simulink model "visual_line_follower_with_debug_real"  (R2026a)
settings: Solver=FixedStepDiscrete  StopTime=inf  FixedStep=Ts_Control  EnableMultiTasking=on
InitFcn:
  | run(fullfile(fileparts(get_param(bdroot,"FileName")),"runtime","init","configure_visual_line_follower_real_debug.m"));
model workspace (MAT data in the model file):
  BaseLinearSpeed = 5
  BaseSpeedScale = 0.03
  Kd_Line = 0.35
  Ki_Line = 0
  Kp_Line = 5
  LocalPath_CurvatureGain = 0.04
  LocalPath_HeadingGain = 0.35
  LocalPath_LateralGain = 0.6
  LocalPath_LookaheadDistance = 0.2
  LocalPath_NumPoints = 30
  LocalPath_ROIFraction = 0.1
  MJ_StepTime = 0.002
  MJ_TargetLateralPosition = 0
  MaxAngularSpeed = 1.5
  MaxWheelSpeed = 7.9
  N_Line = 20
  OriginBot_ErrorScale = 500
  OriginBot_MaxSaturation = 0.3
  OriginBot_MinBrightness = 70
  OriginBot_MinPixels = 30
  OriginBot_ROIHeight = 45
  OriginBot_ROIStartFraction = 0.72
  SL_ROS_VariableLengthArrays_MaxSizes.CommonInfo.ArrayTruncateAction = 'EmitWarning'
  SL_ROS_VariableLengthArrays_MaxSizes.MsgTypeMap = containers.Map
  SL_ROS_VariableLengthArrays_MaxSizes.MsgTypeMap.serialization.keys = {'sensor_msgs/Image'}
  SL_ROS_VariableLengthArrays_MaxSizes.MsgTypeMap.serialization.values{1}(1).PropertyName = 'data'
  SL_ROS_VariableLengthArrays_MaxSizes.MsgTypeMap.serialization.values{1}(1).DataType = 'uint8'
  SL_ROS_VariableLengthArrays_MaxSizes.MsgTypeMap.serialization.values{1}(1).MaxLength = 6220800
  SL_ROS_VariableLengthArrays_MaxSizes.MsgTypeMap.serialization.values{1}(2).PropertyName = 'encoding'
  SL_ROS_VariableLengthArrays_MaxSizes.MsgTypeMap.serialization.values{1}(2).DataType = 'uint8'
  SL_ROS_VariableLengthArrays_MaxSizes.MsgTypeMap.serialization.values{1}(2).MaxLength = 128
  SL_ROS_VariableLengthArrays_MaxSizes.MsgTypeMap.serialization.uniformity = 0
  SL_ROS_VariableLengthArrays_MaxSizes.MsgTypeMap.serialization.keyType = 'char'
  SL_ROS_VariableLengthArrays_MaxSizes.MsgTypeMap.serialization.valueType = 'any'
  SteeringSign = 1
  TB3_WheelRadius = 0.033
  TB3_WheelSeparation = 0.16
  Ts_Control = 0.05
  Ts_Vision = 0.05
  TurtleBot3MuJoCoMap = 'simple'
  TurtleBot3MuJoCoScene = ""
  k_heading = 0.55
undefined symbols (not defined in the file or in its folder): originbot_line_follower_debug_frame, originbot_sliding_window_path_generator, twist
libraries: ros2lib x4, slpidlib x1
settings Model: ExtModeTrigDuration=10000  Creator=HP  LastModifiedBy=kevin
settings SolverCC: PositivePriorityOrder=on
settings ConfigComp: CovMetricSettings=dswe

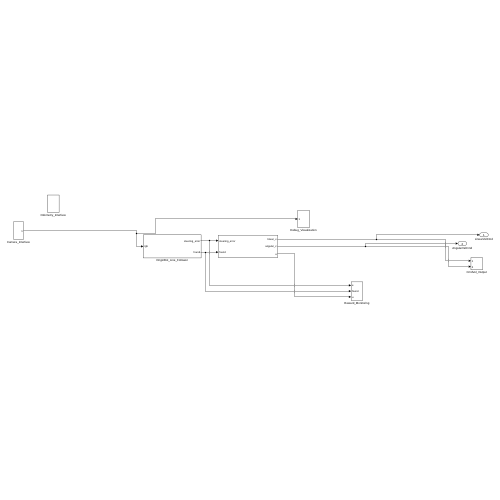
[thumbnail: Simulink's stored preview of the top-level diagram]
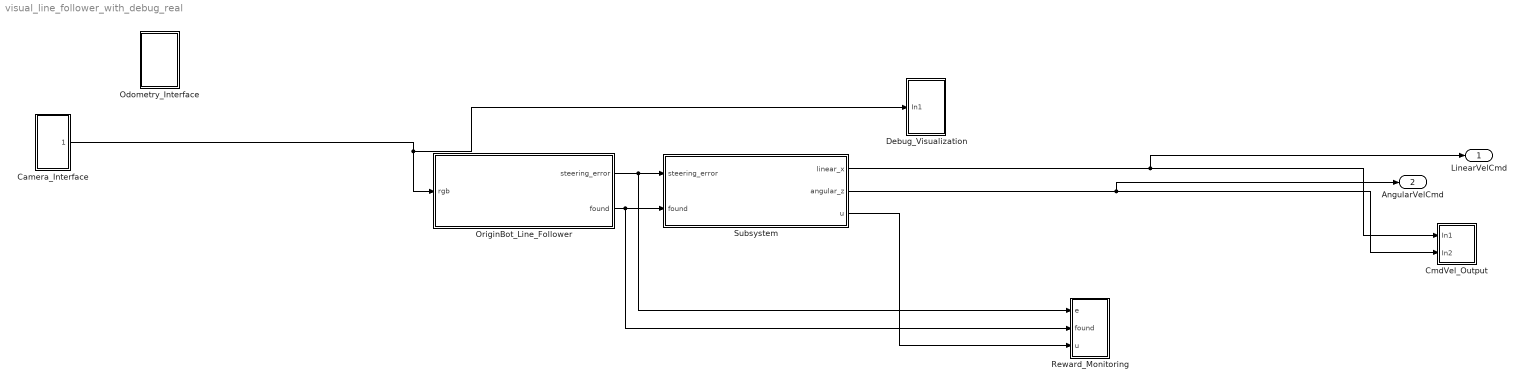
== system visual_line_follower_with_debug_real ==
  Camera_Interface : Subsystem
  CmdVel_Output : Subsystem
  Debug_Visualization : Subsystem
  Odometry_Interface : Subsystem
  OriginBot_Line_Follower : Subsystem
  Reward_Monitoring : Subsystem
  Subsystem : Subsystem
  LinearVelCmd : Outport
  AngularVelCmd : Outport  Port=2
  wires:
  Subsystem/1(linear_x) -> CmdVel_Output/1(In1), LinearVelCmd/1
  Subsystem/2(angular_z) -> CmdVel_Output/2(In2), AngularVelCmd/1
  OriginBot_Line_Follower/1(steering_error) -> Reward_Monitoring/1(e), Subsystem/1(steering_error)
  OriginBot_Line_Follower/2(found) -> Reward_Monitoring/2(found), Subsystem/2(found)
  Camera_Interface/1(Out1) -> Debug_Visualization/1(In1), OriginBot_Line_Follower/1(rgb)
  Subsystem/3(u) -> Reward_Monitoring/3(u)

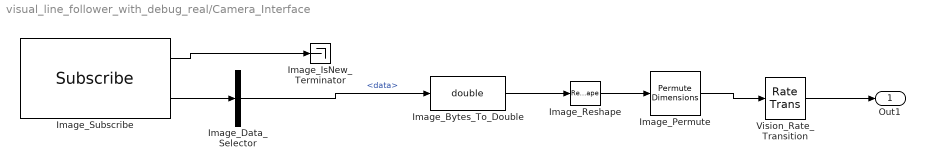
== system visual_line_follower_with_debug_real/Camera_Interface ==
  Image_Bytes_To_Double : DataTypeConversion  OutDataTypeStr=double
  Image_Data_Selector : BusSelector  OutputSignals=data
  Image_IsNew_Terminator : Terminator
  Image_Permute : PermuteDimensions  Order=[3 2 1]
  Image_Reshape : Reshape  OutputDimensionality=Customize  OutputDimensions=[3,1920,1080]
  Image_Subscribe : ros2lib/Subscribe  topicSource=Select from ROS network  topic=/camera/image_raw  messageType=sensor_msgs/Image  sampleTime=Ts_Vision  QOSHistory=Keep last  QOSDepth=10  QOSReliability=Reliable  QOSDurability=Volatile  QOSDeadline=Inf  QOSLifespan=Inf  QOSLiveliness=Automatic  QOSLeaseDuration=Inf  QOSAvoidROSNamespaceConventions=off
  Vision_Rate_Transition : RateTransition
  Out1 : Outport
  wires:
  Image_Permute/1 -> Vision_Rate_Transition/1
  Image_Subscribe/2 -> Image_Data_Selector/1
  Image_Subscribe/1 -> Image_IsNew_Terminator/1
  Image_Data_Selector/1 -> Image_Bytes_To_Double/1  "<data>"
  Vision_Rate_Transition/1 -> Out1/1
  Image_Bytes_To_Double/1 -> Image_Reshape/1
  Image_Reshape/1 -> Image_Permute/1

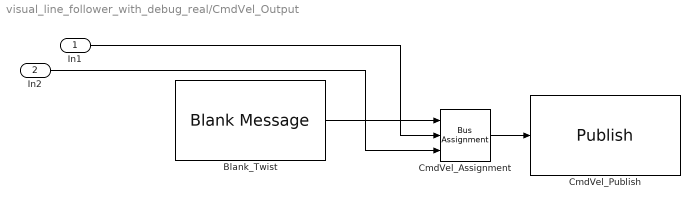
== system visual_line_follower_with_debug_real/CmdVel_Output ==
  In1 : Inport
  In2 : Inport  Port=2
  Blank_Twist : ros2lib/Blank Message  messageClass=Message  entityType=geometry_msgs/TwistStamped  messageType=geometry_msgs/TwistStamped  SampleTime=inf
  CmdVel_Assignment : BusAssignment  AssignedSignals=twist.linear.x,twist.angular.z
  CmdVel_Publish : ros2lib/Publish  topicSource=Select from ROS network  topic=/cmd_vel  messageType=geometry_msgs/TwistStamped  QOSHistory=Keep last  QOSDepth=10  QOSReliability=Reliable  QOSDurability=Volatile  QOSDeadline=Inf  QOSLifespan=Inf  QOSLiveliness=Automatic  QOSLeaseDuration=Inf  QOSAvoidROSNamespaceConventions=off
  wires:
  In2/1 -> CmdVel_Assignment/3
  Blank_Twist/1 -> CmdVel_Assignment/1
  CmdVel_Assignment/1 -> CmdVel_Publish/1
  In1/1 -> CmdVel_Assignment/2

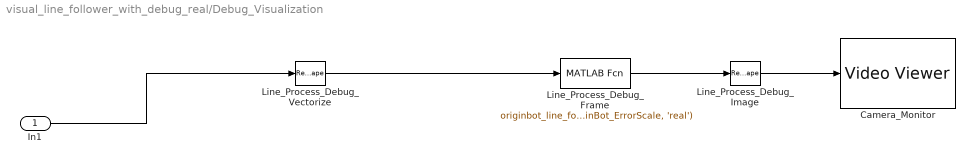
== system visual_line_follower_with_debug_real/Debug_Visualization ==
  In1 : Inport
  Camera_Monitor : VideoViewer  FigPos=[751 777 651 427]
  Line_Process_Debug_Frame : MATLABFcn  MATLABFcn=originbot_line_follower_debug_frame(u, LocalPath_ROIFraction, LocalPath_NumPoints, OriginBot_MinBrightness, OriginBot_MaxSaturation, OriginBot_MinPixels, OriginBot_ErrorScale, 'real')
  Line_Process_Debug_Image : Reshape  OutputDimensionality=Customize  OutputDimensions=[1080,1920,3]
  Line_Process_Debug_Vectorize : Reshape  OutputDimensionality=Column vector (2-D)
  wires:
  Line_Process_Debug_Vectorize/1 -> Line_Process_Debug_Frame/1
  Line_Process_Debug_Image/1 -> Camera_Monitor/1
  Line_Process_Debug_Frame/1 -> Line_Process_Debug_Image/1
  In1/1 -> Line_Process_Debug_Vectorize/1

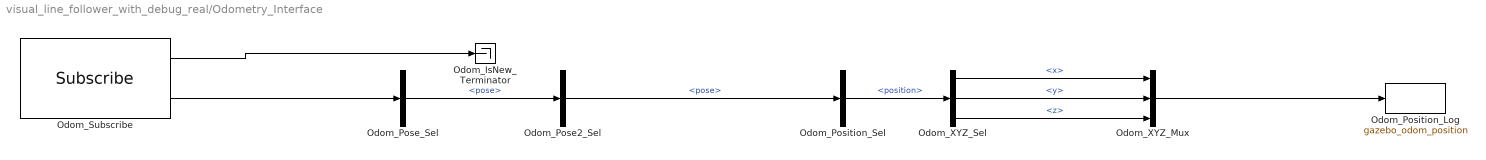
== system visual_line_follower_with_debug_real/Odometry_Interface ==
  Odom_IsNew_Terminator : Terminator
  Odom_Pose2_Sel : BusSelector  OutputSignals=pose
  Odom_Pose_Sel : BusSelector  OutputSignals=pose
  Odom_Position_Log : ToWorkspace  VariableName=gazebo_odom_position  SaveFormat=Timeseries  SampleTime=-1
  Odom_Position_Sel : BusSelector  OutputSignals=position
  Odom_Subscribe : ros2lib/Subscribe  topicSource=Select from ROS network  topic=/odom  messageType=nav_msgs/Odometry  sampleTime=Ts_Control  QOSHistory=Keep last  QOSDepth=10  QOSReliability=Reliable  QOSDurability=Volatile  QOSDeadline=Inf  QOSLifespan=Inf  QOSLiveliness=Automatic  QOSLeaseDuration=Inf  QOSAvoidROSNamespaceConventions=off
  Odom_XYZ_Mux : Mux  Inputs=3
  Odom_XYZ_Sel : BusSelector  OutputSignals=x,y,z
  wires:
  Odom_Subscribe/1 -> Odom_IsNew_Terminator/1
  Odom_XYZ_Sel/3 -> Odom_XYZ_Mux/3  "<z>"
  Odom_Position_Sel/1 -> Odom_XYZ_Sel/1  "<position>"
  Odom_XYZ_Sel/1 -> Odom_XYZ_Mux/1  "<x>"
  Odom_XYZ_Sel/2 -> Odom_XYZ_Mux/2  "<y>"
  Odom_Pose_Sel/1 -> Odom_Pose2_Sel/1  "<pose>"
  Odom_Subscribe/2 -> Odom_Pose_Sel/1
  Odom_Pose2_Sel/1 -> Odom_Position_Sel/1  "<pose>"
  Odom_XYZ_Mux/1 -> Odom_Position_Log/1

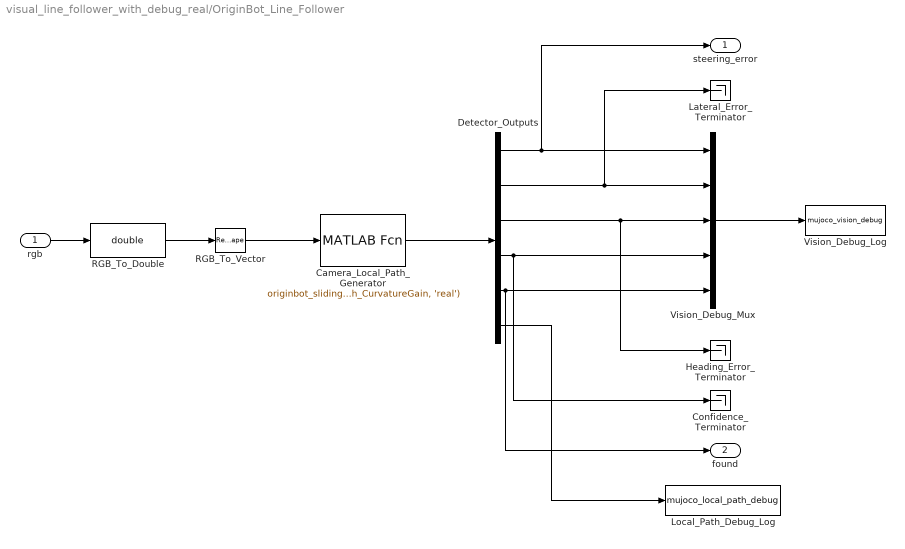
== system visual_line_follower_with_debug_real/OriginBot_Line_Follower ==
  rgb : Inport
  Camera_Local_Path_Generator : MATLABFcn  MATLABFcn=originbot_sliding_window_path_generator(u, LocalPath_ROIFraction, LocalPath_NumPoints, OriginBot_MinBrightness, OriginBot_MaxSaturation, OriginBot_MinPixels, OriginBot_ErrorScale, LocalPath_LookaheadDistance, LocalPath_LateralGain, LocalPath_HeadingGain, LocalPath_CurvatureGain, 'real')  OutputDimensions=72  OutputSignalType=real  SampleTime=Ts_Vision
  Confidence_Terminator : Terminator
  Detector_Outputs : Demux  Outputs=[1 1 1 1 1 67]
  Heading_Error_Terminator : Terminator
  Lateral_Error_Terminator : Terminator
  Local_Path_Debug_Log : ToWorkspace  VariableName=mujoco_local_path_debug  SaveFormat=Timeseries  SampleTime=-1
  RGB_To_Double : DataTypeConversion  OutDataTypeStr=double
  RGB_To_Vector : Reshape  OutputDimensionality=Column vector (2-D)
  Vision_Debug_Log : ToWorkspace  VariableName=mujoco_vision_debug  SaveFormat=Timeseries  SampleTime=-1
  Vision_Debug_Mux : Mux  Inputs=5
  steering_error : Outport
  found : Outport  Port=2
  wires:
  Vision_Debug_Mux/1 -> Vision_Debug_Log/1
  Detector_Outputs/1 -> steering_error/1, Vision_Debug_Mux/1
  Detector_Outputs/5 -> Vision_Debug_Mux/5, found/1
  Detector_Outputs/2 -> Vision_Debug_Mux/2, Lateral_Error_Terminator/1
  Detector_Outputs/6 -> Local_Path_Debug_Log/1
  Detector_Outputs/3 -> Vision_Debug_Mux/3, Heading_Error_Terminator/1
  Detector_Outputs/4 -> Confidence_Terminator/1, Vision_Debug_Mux/4
  RGB_To_Double/1 -> RGB_To_Vector/1
  RGB_To_Vector/1 -> Camera_Local_Path_Generator/1
  rgb/1 -> RGB_To_Double/1
  Camera_Local_Path_Generator/1 -> Detector_Outputs/1

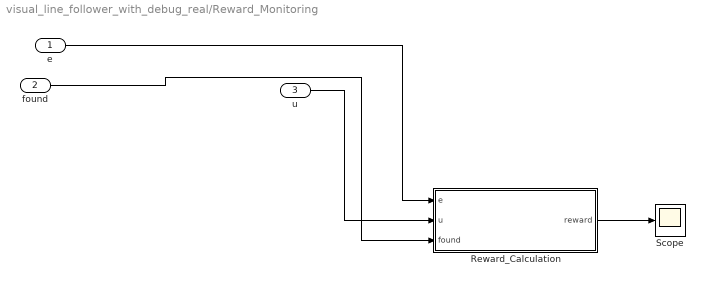
== system visual_line_follower_with_debug_real/Reward_Monitoring ==
  e : Inport
  found : Inport  Port=2
  u : Inport  Port=3
  Reward_Calculation : Subsystem
  Scope : Scope
      settings: ActiveDisplayYMinimum=-19.654077355148576  ActiveDisplayYMaximum=1.5094488795252738
  wires:
  Reward_Calculation/1(reward) -> Scope/1
  u/1 -> Reward_Calculation/2(u)
  e/1 -> Reward_Calculation/1(e)
  found/1 -> Reward_Calculation/3(found)

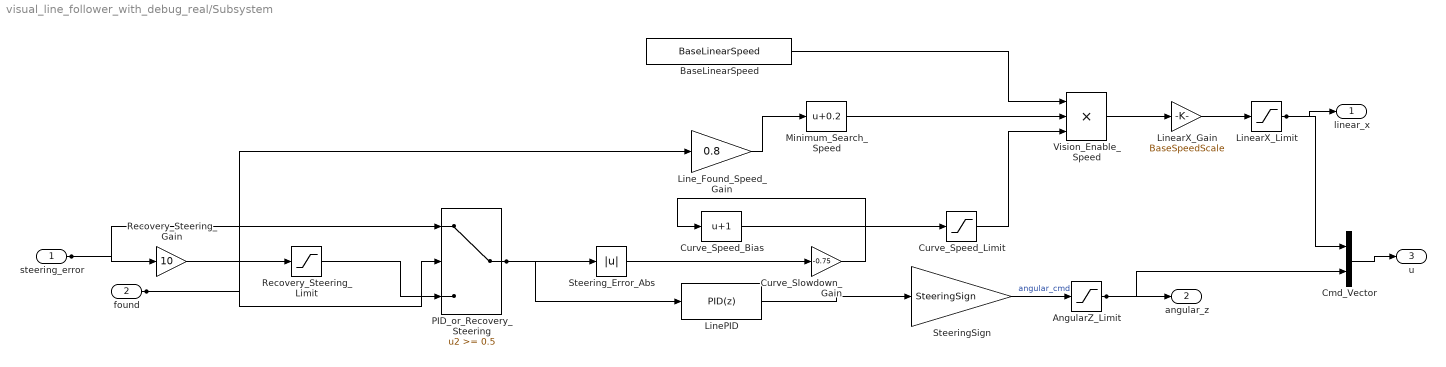
== system visual_line_follower_with_debug_real/Subsystem ==
  steering_error : Inport
  found : Inport  Port=2
  AngularZ_Limit : Saturate  UpperLimit=2*MaxWheelSpeed*TB3_WheelRadius/TB3_WheelSeparation  LowerLimit=-2*MaxWheelSpeed*TB3_WheelRadius/TB3_WheelSeparation
  BaseLinearSpeed : Constant  Value=BaseLinearSpeed
  Cmd_Vector : Mux  Inputs=2
  Curve_Slowdown_Gain : Gain  Gain=-0.75
  Curve_Speed_Bias : Bias  Bias=1
  Curve_Speed_Limit : Saturate  UpperLimit=1  LowerLimit=0.25
  LinePID : slpidlib/PID Controller  Controller=PID  Form=Parallel  TimeDomain=Discrete-time  UseExternalTs=off  SampleTime=Ts_Control  IntegratorMethod=Backward Euler  FilterMethod=Trapezoidal  ControllerParametersSource=internal  P=Kp_Line  I=Ki_Line  UseKiTs=off  D=Kd_Line  UseExternalDerivativeSource=off  N=N_Line  UseFilter=on  TunerSelectOption=Transfer Function Based (PID Tuner App)  InitialConditionSource=internal  InitialConditionForIntegrator=0  InitialConditionForFilter=0  DifferentiatorICPrevScaledInput=0  ExternalReset=none  TrackingMode=off  Kt=1  LimitOutput=on  SatLimitsSource=internal  UpperSaturationLimit=MaxAngularSpeed  LowerSaturationLimit=-MaxAngularSpeed  LinearizeAsGain=off  AntiWindupMode=back-calculation  Kb=1  LimitIntegrator=off  UpperIntegratorSaturationLimit=inf  LowerIntegratorSaturationLimit=-inf  POutMin=[]  POutMax=[]  IOutMin=[]  IOutMax=[]  DOutMin=[]  DOutMax=[]  NOutMin=[]  NOutMax=[]  SumOutMin=[]  SumOutMax=[]  SaturationOutMin=[]  SaturationOutMax=[]  PParamMin=[]  PParamMax=[]  IParamMin=[]  IParamMax=[]  DParamMin=[]  DParamMax=[]  NParamMin=[]  NParamMax=[]  KbParamMin=[]  KbParamMax=[]  KtParamMin=[]  KtParamMax=[]  KbOutMin=[]  KbOutMax=[]  KtOutMin=[]  KtOutMax=[]  IntegratorOutMin=[]  IntegratorOutMax=[]  FilterOutMin=[]  FilterOutMax=[]  SumI1OutMin=[]  SumI1OutMax=[]  SumI2OutMin=[]  SumI2OutMax=[]  SumI3OutMin=[]  SumI3OutMax=[]  SumI4OutMin=[]  SumI4OutMax=[]  SumDOutMin=[]  SumDOutMax=[]  DifferentiatorOutMin=[]  DifferentiatorOutMax=[]  FilterDiffOutCoefMin=[]  FilterDiffOutCoefMax=[]  ReciprocalOutMin=[]  ReciprocalOutMax=[]  SumDenOutMin=[]  SumDenOutMax=[]  SumNumOutMin=[]  SumNumOutMax=[]  DivideOutMin=[]  DivideOutMax=[]  UdiffTsProdOutMin=[]  UdiffTsProdOutMax=[]  NTsProdOutMin=[]  NTsProdOutMax=[]  UintegralTsProdOutMin=[]  UintegralTsProdOutMax=[]  UngainTsProdOutMin=[]  UngainTsProdOutMax=[]  ClampingZeroOutDataTypeStr=Inherit: Inherit via back propagation  ClampingZeroOutMin=[]  ClampingZeroOutMax=[]  FilterDenConstantOutDataTypeStr=Inherit: Inherit via back propagation  FilterDenConstantOutMin=[]  FilterDenConstantOutMax=[]  PCopyOutDataTypeStr=Inherit: Inherit via back propagation  PCopyOutMin=[]  PCopyOutMax=[]  NCopyOutDataTypeStr=Inherit: Inherit via back propagation  NCopyOutMin=[]  NCopyOutMax=[]  IntegratorContinuousStateAttributes=''  IntegratorStateMustResolveToSignalObject=off  IntegratorRTWStateStorageClass=Auto  FilterContinuousStateAttributes=''  FilterStateMustResolveToSignalObject=off  FilterRTWStateStorageClass=Auto  ParallelPVariant=InternalParameters  IdealPVariant=Disabled  IVariant=InternalParameters  DVariant=InternalParameters  IntegratorVariant=Discrete  SatVariant=Enabled  AWVariant=BackCalculation  PCopyVariant=Disabled  TRVariant=Disabled  FdbkBlocksVariant=Feedback  IdealPFdbkVariant=Passthrough  SatFdbkVariant=Enabled  DerivativeFilterVariant=TrapezoidalFilter  NVariant=InternalParameters  NCopyVariant=InternalParameters  FilterICVariant=InternalICsFilter  IntegratorICVariant=InternalICs  ExternalResetVariant=Disabled  TRSumVariant=Passthrough  SumFdbkVariant=Enabled  SumVariant=Sum_PID  TsampFilterVariant=InternalTs  TsampNgainVariant=Passthrough  TsampIntegralVariant=Disabled_SignalSpec  ExternalSaturationOutDataTypeStr=Inherit: Same as second input  DerivativeSourceVariant=ErrorSignal  PreIntVariant=InternalPreInt
      settings: LibrarySourceBlock=hdlsllib/Discrete/Discrete PID Controller
  Line_Found_Speed_Gain : Gain  Gain=0.8
  LinearX_Gain : Gain  Gain=BaseSpeedScale
  LinearX_Limit : Saturate  UpperLimit=MaxWheelSpeed*TB3_WheelRadius  LowerLimit=-MaxWheelSpeed*TB3_WheelRadius
  Minimum_Search_Speed : Bias  Bias=0.2
  PID_or_Recovery_Steering : Switch  Threshold=0.5
  Recovery_Steering_Gain : Gain  Gain=10
  Recovery_Steering_Limit : Saturate  UpperLimit=0.45  LowerLimit=-0.45
  SteeringSign : Gain  Gain=SteeringSign
  Steering_Error_Abs : Abs
  Vision_Enable_Speed : Product  Inputs=***
  linear_x : Outport
  angular_z : Outport  Port=2
  u : Outport  Port=3
  wires:
  Cmd_Vector/1 -> u/1
  AngularZ_Limit/1 -> Cmd_Vector/2, angular_z/1
  SteeringSign/1 -> AngularZ_Limit/1  "angular_cmd"
  LinearX_Limit/1 -> linear_x/1, Cmd_Vector/1
  LinearX_Gain/1 -> LinearX_Limit/1
  Vision_Enable_Speed/1 -> LinearX_Gain/1
  Curve_Speed_Limit/1 -> Vision_Enable_Speed/3
  BaseLinearSpeed/1 -> Vision_Enable_Speed/1
  LinePID/1 -> SteeringSign/1
  Curve_Speed_Bias/1 -> Curve_Speed_Limit/1
  Curve_Slowdown_Gain/1 -> Curve_Speed_Bias/1
  Steering_Error_Abs/1 -> Curve_Slowdown_Gain/1
  Line_Found_Speed_Gain/1 -> Minimum_Search_Speed/1
  Recovery_Steering_Limit/1 -> PID_or_Recovery_Steering/3
  Recovery_Steering_Gain/1 -> Recovery_Steering_Limit/1
  PID_or_Recovery_Steering/1 -> LinePID/1, Steering_Error_Abs/1
  found/1 -> PID_or_Recovery_Steering/2, Line_Found_Speed_Gain/1
  Minimum_Search_Speed/1 -> Vision_Enable_Speed/2
  steering_error/1 -> Recovery_Steering_Gain/1, PID_or_Recovery_Steering/1

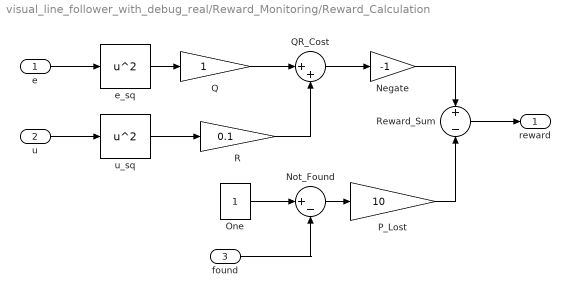
== system visual_line_follower_with_debug_real/Reward_Monitoring/Reward_Calculation ==
  e : Inport
  u : Inport  Port=2
  found : Inport  Port=3
  Negate : Gain  Gain=-1
  Not_Found : Sum  Inputs=|+-
  One : Constant
  P_Lost : Gain  Gain=10
  Q : Gain
  QR_Cost : Sum  Inputs=|++
  R : Gain  Gain=0.1
  Reward_Sum : Sum  Inputs=+-
  e_sq : Math  Operator=square
  u_sq : Math  Operator=square
  reward : Outport
  wires:
  Q/1 -> QR_Cost/1
  e/1 -> e_sq/1
  u/1 -> u_sq/1
  R/1 -> QR_Cost/2
  e_sq/1 -> Q/1
  u_sq/1 -> R/1
  One/1 -> Not_Found/1
  found/1 -> Not_Found/2
  QR_Cost/1 -> Negate/1
  Not_Found/1 -> P_Lost/1
  P_Lost/1 -> Reward_Sum/2
  Negate/1 -> Reward_Sum/1
  Reward_Sum/1 -> reward/1
